simulink model "upr_1_1"  (R2019a)
settings: Solver=FixedStepAuto  StartTime=0.0  StopTime=100  FixedStep=Ts  RelTol=1e-3
values from neighbouring files (symbols this model uses):
  Kp = 1    [1upr.m]    (also in upr_1.m)
  Kp_pos = Kp/2*(1+sqrt(1-4*Td/Ti))    [upr_1.m]
  Td = 3    [1upr.m]    (also in PIDtun_CC.m = L*(0.37-0.37*tau)/(1-0.81*tau); PIDtun_ZN1.m = L/2; PIDtun_ZN2.m = 0.125*Tu; upr_1.m = 0.04)
  Td_pos = Td/2*(1+sqrt(1-4*Td/Ti))    [upr_1.m]
  Ti = 0.5    [1upr.m]    (also in PIDtun_CC.m = L*(2.5-2*tau)/(1-0.39*tau); PIDtun_ZN1.m = 2*L; PIDtun_ZN2.m = 0.5*Tu; upr_1.m = 0.2)
  Ti_pos = Ti/2*(1+sqrt(1-4*Td/Ti))    [upr_1.m]
settings Model: Creator=user1  LastModifiedBy=user1

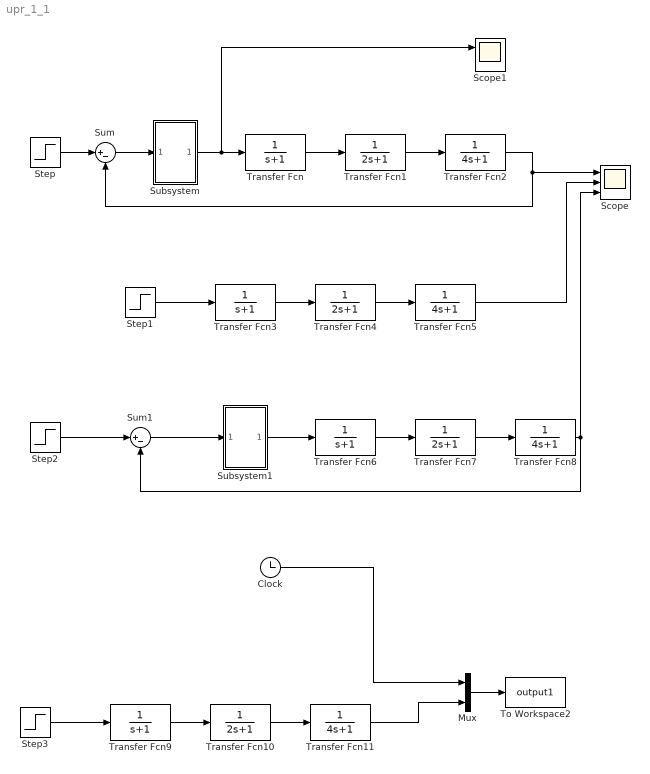
== system upr_1_1 ==
  Clock : Clock
  Mux : Mux  Inputs=2
  Scope : Scope  NumInputPorts=3
  Scope1 : Scope  NumInputPorts=2
  Step{,1..3} (4 alike) : Step  SampleTime=0
  Subsystem : Subsystem
  Subsystem1 : Subsystem
  Sum : Sum  Inputs=|+-
  Sum1 : Sum  Inputs=|+-
  To Workspace2 : ToWorkspace  VariableName=output1  SampleTime=-1
      settings: Save2DSignal=2-D array (concatenate along first dimension)
  Transfer Fcn{,3,6,9} (4 alike) : TransferFcn  Denominator=[1 1]
  Transfer Fcn{1,4,7,10} (4 alike) : TransferFcn  Denominator=[2 1]
  Transfer Fcn{2,5,8,11} (4 alike) : TransferFcn  Denominator=[4 1]
  wires:
  Step/1 -> Sum/1
  Sum/1 -> Subsystem/1(In1)
  Subsystem/1(Out1) -> Scope1/1, Transfer Fcn/1
  Transfer Fcn1/1 -> Transfer Fcn2/1
  Transfer Fcn2/1 -> Sum/2, Scope/1
  Transfer Fcn/1 -> Transfer Fcn1/1
  Transfer Fcn4/1 -> Transfer Fcn5/1
  Transfer Fcn3/1 -> Transfer Fcn4/1
  Step1/1 -> Transfer Fcn3/1
  Transfer Fcn5/1 -> Scope/2
  Transfer Fcn6/1 -> Transfer Fcn7/1
  Transfer Fcn7/1 -> Transfer Fcn8/1
  Subsystem1/1(Out1) -> Transfer Fcn6/1
  Sum1/1 -> Subsystem1/1(In1)
  Step2/1 -> Sum1/1
  Transfer Fcn8/1 -> Scope/3, Sum1/2
  Clock/1 -> Mux/1
  Step3/1 -> Transfer Fcn9/1
  Transfer Fcn10/1 -> Transfer Fcn11/1
  Transfer Fcn9/1 -> Transfer Fcn10/1
  Mux/1 -> To Workspace2/1
  Transfer Fcn11/1 -> Mux/2

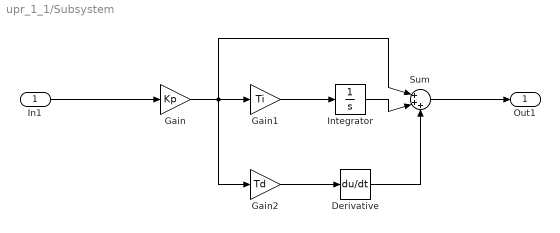
== system upr_1_1/Subsystem ==
  In1 : Inport
  Derivative : Derivative
  Gain : Gain  Gain=Kp
  Gain1 : Gain  Gain=Ti
  Gain2 : Gain  Gain=Td
  Integrator : Integrator
  Sum : Sum  Inputs=|+++
  Out1 : Outport
  wires:
  Gain1/1 -> Integrator/1
  Sum/1 -> Out1/1
  Gain/1 -> Sum/1, Gain2/1, Gain1/1
  In1/1 -> Gain/1
  Derivative/1 -> Sum/3
  Integrator/1 -> Sum/2
  Gain2/1 -> Derivative/1

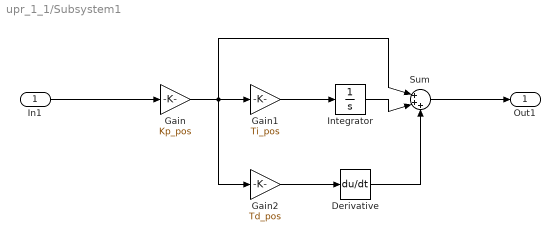
== system upr_1_1/Subsystem1 ==
  In1 : Inport
  Derivative : Derivative
  Gain : Gain  Gain=Kp_pos
  Gain1 : Gain  Gain=Ti_pos
  Gain2 : Gain  Gain=Td_pos
  Integrator : Integrator
  Sum : Sum  Inputs=|+++
  Out1 : Outport
  wires:
  Gain1/1 -> Integrator/1
  Sum/1 -> Out1/1
  Gain/1 -> Sum/1, Gain2/1, Gain1/1
  In1/1 -> Gain/1
  Derivative/1 -> Sum/3
  Integrator/1 -> Sum/2
  Gain2/1 -> Derivative/1
